simulink model "RLSUpdate_th"  (R2018a)
settings: Solver=FixedStepDiscrete  StartTime=0.0  StopTime=100  FixedStep=0.25  RelTol=1e-3
undefined symbols (not defined in the file or in its folder): p
libraries: RLSUpdate_ul x1
settings Model: Creator=mitch  LastModifiedBy=mitch

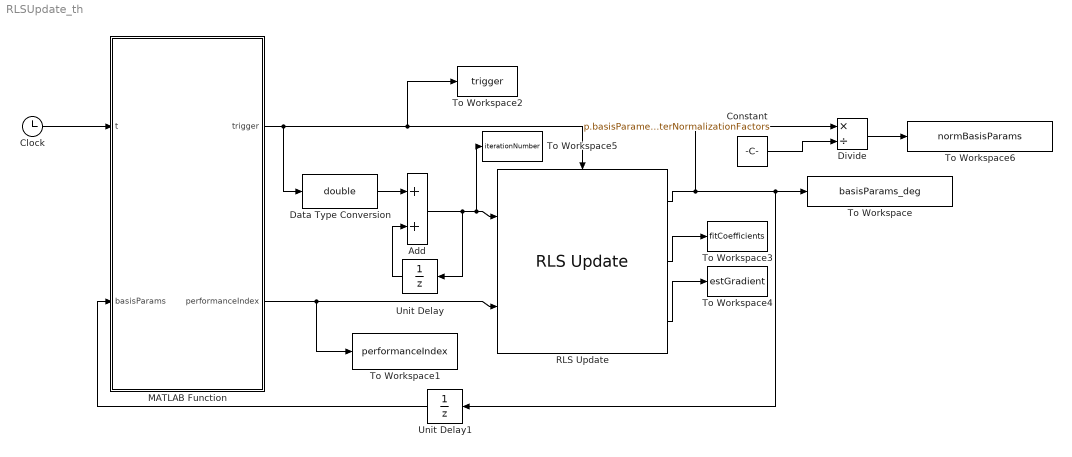
== system RLSUpdate_th ==
  Add : Sum
  Clock : Clock
  Constant : Constant  Value=p.basisParameterNormalizationFactors
  Data Type Conversion : DataTypeConversion  OutDataTypeStr=double
  Divide : Product  Inputs=*/
  MATLAB Function : MATLAB Function  TreatAsAtomicUnit=on
  RLS Update : RLSUpdate_ul/RLS Update  settlingBasisParameter=[p.width p.height]'  initializationBasisParameters=p.initializationBasisParameters  numSettlingLaps=p.numSettlingLaps  forgettingFactor=p.forgettingFactor  normalizationFactors=p.basisParameterNormalizationFactors'  trustRegionDimensions=p.trustRegionDimensions'  learningGain=p.KLearningGradient  noiseAmplitude=0
  To Workspace : ToWorkspace  VariableName=basisParams_deg  SaveFormat=Timeseries  SampleTime=-1
  To Workspace1 : ToWorkspace  VariableName=performanceIndex  SaveFormat=Timeseries  SampleTime=-1
  To Workspace2 : ToWorkspace  VariableName=trigger  SaveFormat=Timeseries  SampleTime=-1
  To Workspace3 : ToWorkspace  VariableName=fitCoefficients  SaveFormat=Timeseries  SampleTime=-1
  To Workspace4 : ToWorkspace  VariableName=estGradient  SaveFormat=Timeseries  SampleTime=-1
  To Workspace5 : ToWorkspace  VariableName=iterationNumber  SaveFormat=Timeseries  SampleTime=-1
  To Workspace6 : ToWorkspace  VariableName=normBasisParams  SaveFormat=Timeseries  SampleTime=-1
  Unit Delay : UnitDelay  InitialCondition=-1  SampleTime=-1
  Unit Delay1 : UnitDelay  InitialCondition=[p.width p.height]  SampleTime=-1
  wires:
  Clock/1 -> MATLAB Function/1(t)
  MATLAB Function/1(trigger) -> Data Type Conversion/1, RLS Update/Trigger, To Workspace2/1
  MATLAB Function/2(performanceIndex) -> To Workspace1/1, RLS Update/2
  Add/1 -> To Workspace5/1, RLS Update/1, Unit Delay/1
  Unit Delay/1 -> Add/2
  Data Type Conversion/1 -> Add/1
  Unit Delay1/1 -> MATLAB Function/2(basisParams)
  RLS Update/2 -> To Workspace3/1
  RLS Update/3 -> To Workspace4/1
  RLS Update/1 -> Divide/1, Unit Delay1/1, To Workspace/1
  Divide/1 -> To Workspace6/1
  Constant/1 -> Divide/2

== matlab function RLSUpdate_th/MATLAB Function ==
  data: t input; trigger output; basisParams input; performanceIndex output
function [trigger,performanceIndex] = fcn(t,basisParams)

trigger = false;
if rem(t,1)==0
    trigger = true;
end
performanceIndex = truePerformanceIndex(basisParams(1),basisParams(2));
end
